simulink library "libMdl_ImuDataCorrector"  (R2019b)
settings: Solver=VariableStepAuto  StartTime=0.0  StopTime=10.0  RelTol=1e-3
undefined symbols (not defined in the file): f_euler_ma_time, imu_lever_arm, sample_time
libraries: libMdl_transformVect x2, libMdl_crossProdMat x2, simulink x1
settings Model: Creator=Hanno  LastModifiedBy=wint_hn

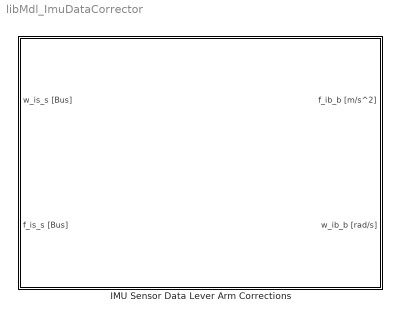
== system libMdl_ImuDataCorrector ==
  IMU Sensor Data Lever Arm Corrections : Subsystem  TreatAsAtomicUnit=on  SystemSampleTime=mv_sample_time  mask(IMU Sensor Data Corrections){mv_lever_arm=imu_lever_arm, mv_mounting_attitude=[1;0;0;0], mv_enable_euler_correction=on, mv_euler_ma_time=f_euler_ma_time, mv_sample_time=sample_time}
      mask prompts: mv_lever_arm "Lever Arm:"; mv_mounting_attitude "Mounting Attitude:"; mv_enable_euler_correction "Enable Euler Correction"; mv_euler_ma_time "Moving Av. Window for Euler Correction:"; mv_sample_time "Sample Time:"
      mask help:
      | Lever Arm: Lever Arm Vector 'leverarm_s_b' in meters describing the mounting position of the sensor with respect to the body frame.
      |
      | Mountin Attitude: Quaternion 'q_s_b' describing the mounting attitude of the sensor with respect to the body frame.
      mask Display:
      | if mv_enable_euler_correction
      |     euler_str = 'on';
      | else
      |     euler_str = 'off';
      | end % if
      | 
      | str1 = sprintf('\\color{black}{\\bfIMU Data Correction}\n\n');
      | str2 = sprintf('Euler Correction: %s\n',euler_str);
      | str3 = sprintf('Euler MA Time: %0.2f\n',mv_euler_ma_time);
      | str4 = sprintf('Sample Time: %0.3f',mv_sample_time);
      | 
      | str = [str1,str2,str3,str4];
      | 
      | text( 0.5,0.5, ...
      |       str, ...
      |       'horizontalAlignment', 'center', ...
      |       'texmode','on' ...
      |     )

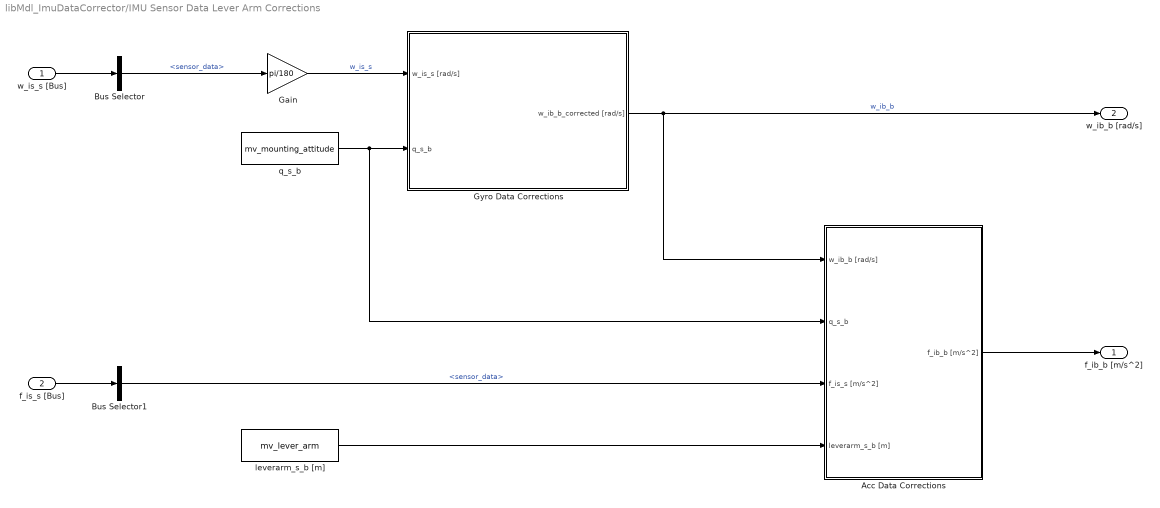
== system libMdl_ImuDataCorrector/IMU Sensor Data Lever Arm Corrections ==
  w_is_s [Bus] : Inport
  f_is_s [Bus] : Inport  Port=2
  Acc Data Corrections : Subsystem
  Bus Selector : BusSelector  OutputSignals=sensor_data
  Bus Selector1 : BusSelector  OutputSignals=sensor_data
  Gain : Gain  Gain=pi/180
      settings: AttributesFormatString=deg2rad
  Gyro Data Corrections : Subsystem
  leverarm_s_b [m] : Constant  Value=mv_lever_arm
  q_s_b : Constant  Value=mv_mounting_attitude
  f_ib_b [m/s^2] : Outport  VectorParamsAs1DForOutWhenUnconnected=off
  w_ib_b [rad/s] : Outport  Port=2  VectorParamsAs1DForOutWhenUnconnected=off
  wires:
  Gyro Data Corrections/1(w_ib_b_corrected [rad/s]) -> w_ib_b [rad/s]/1, Acc Data Corrections/1(w_ib_b [rad/s])  "w_ib_b"
  f_is_s [Bus]/1 -> Bus Selector1/1
  Acc Data Corrections/1(f_ib_b [m/s^2]) -> f_ib_b [m/s^2]/1
  w_is_s [Bus]/1 -> Bus Selector/1
  q_s_b/1 -> Acc Data Corrections/2(q_s_b), Gyro Data Corrections/2(q_s_b)
  leverarm_s_b [m]/1 -> Acc Data Corrections/4(leverarm_s_b [m])
  Bus Selector/1 -> Gain/1  "<sensor_data>"
  Gain/1 -> Gyro Data Corrections/1(w_is_s [rad/s])  "w_is_s"
  Bus Selector1/1 -> Acc Data Corrections/3(f_is_s [m/s^2])  "<sensor_data>"

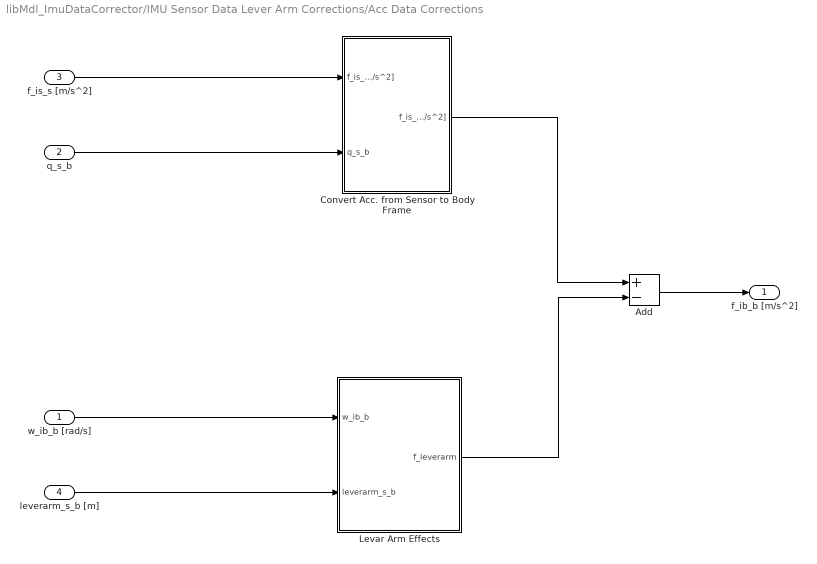
== system libMdl_ImuDataCorrector/IMU Sensor Data Lever Arm Corrections/Acc Data Corrections ==
  w_ib_b [rad/s] : Inport
  q_s_b : Inport  Port=2
  f_is_s [m/s^2] : Inport  Port=3
  leverarm_s_b [m] : Inport  Port=4
  Add : Sum  Inputs=+-
  Convert Acc. from Sensor to Body Frame : Subsystem
  Levar Arm Effects : Subsystem
  f_ib_b [m/s^2] : Outport  VectorParamsAs1DForOutWhenUnconnected=off
  wires:
  Levar Arm Effects/1(f_leverarm) -> Add/2
  f_is_s [m/s^2]/1 -> Convert Acc. from Sensor to Body Frame/1(f_is_s [m/s^2])
  q_s_b/1 -> Convert Acc. from Sensor to Body Frame/2(q_s_b)
  leverarm_s_b [m]/1 -> Levar Arm Effects/2(leverarm_s_b)
  w_ib_b [rad/s]/1 -> Levar Arm Effects/1(w_ib_b)
  Convert Acc. from Sensor to Body Frame/1(f_is_b [m/s^2]) -> Add/1
  Add/1 -> f_ib_b [m/s^2]/1

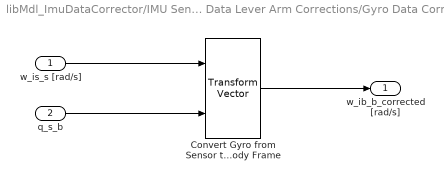
== system libMdl_ImuDataCorrector/IMU Sensor Data Lever Arm Corrections/Gyro Data Corrections ==
  w_is_s [rad/s] : Inport
  q_s_b : Inport  Port=2
  Convert Gyro from Sensor to Body Frame : libMdl_transformVect/Transform Vector  SystemSampleTime=-1  Latency=0  AutoFrameSizeCalculation=off
  w_ib_b_corrected [rad/s] : Outport  VectorParamsAs1DForOutWhenUnconnected=off
  wires:
  Convert Gyro from Sensor to Body Frame/1 -> w_ib_b_corrected [rad/s]/1
  q_s_b/1 -> Convert Gyro from Sensor to Body Frame/2
  w_is_s [rad/s]/1 -> Convert Gyro from Sensor to Body Frame/1

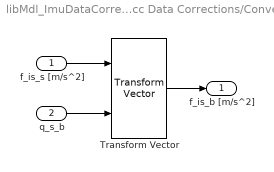
== system libMdl_ImuDataCorrector/IMU Sensor Data Lever Arm Corrections/Acc Data Corrections/Convert Acc. from Sensor to Body Frame ==
  f_is_s [m/s^2] : Inport
  q_s_b : Inport  Port=2
  Transform Vector : libMdl_transformVect/Transform Vector  SystemSampleTime=-1  Latency=0  AutoFrameSizeCalculation=off
  f_is_b [m/s^2] : Outport  VectorParamsAs1DForOutWhenUnconnected=off
  wires:
  f_is_s [m/s^2]/1 -> Transform Vector/1
  q_s_b/1 -> Transform Vector/2
  Transform Vector/1 -> f_is_b [m/s^2]/1

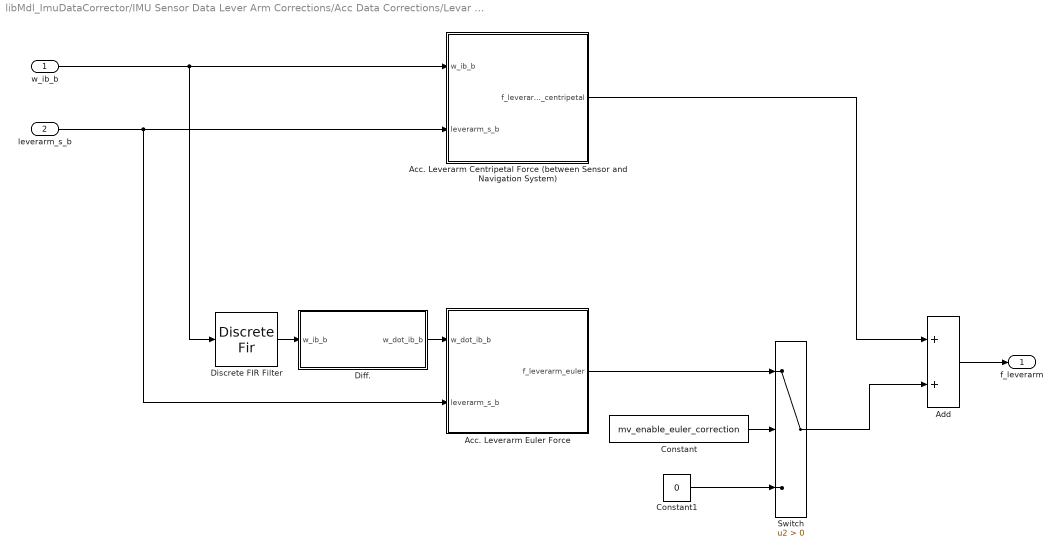
== system libMdl_ImuDataCorrector/IMU Sensor Data Lever Arm Corrections/Acc Data Corrections/Levar Arm Effects ==
  w_ib_b : Inport
  leverarm_s_b : Inport  Port=2
  Acc. Leverarm Centripetal Force (between Sensor and Navigation System) : Subsystem
  Acc. Leverarm Euler Force : Subsystem
  Add : Sum
  Constant : Constant  Value=mv_enable_euler_correction
  Constant1 : Constant  Value=0
  Diff. : Subsystem
  Discrete FIR Filter : DiscreteFir  Coefficients=ones(1,ceil(mv_euler_ma_time/sample_time)) * 1/ceil(mv_euler_ma_time/sample_time)
  Switch : Switch  Criteria=u2 > Threshold
  f_leverarm : Outport  VectorParamsAs1DForOutWhenUnconnected=off
  wires:
  Constant1/1 -> Switch/3
  Acc. Leverarm Euler Force/1(f_leverarm_euler) -> Switch/1
  Constant/1 -> Switch/2
  Switch/1 -> Add/2
  w_ib_b/1 -> Discrete FIR Filter/1, Acc. Leverarm Centripetal Force (between Sensor and Navigation System)/1(w_ib_b)
  Diff./1(w_dot_ib_b) -> Acc. Leverarm Euler Force/1(w_dot_ib_b)
  leverarm_s_b/1 -> Acc. Leverarm Euler Force/2(leverarm_s_b), Acc. Leverarm Centripetal Force (between Sensor and Navigation System)/2(leverarm_s_b)
  Add/1 -> f_leverarm/1
  Acc. Leverarm Centripetal Force (between Sensor and Navigation System)/1(f_leverarm_centripetal) -> Add/1
  Discrete FIR Filter/1 -> Diff./1(w_ib_b)

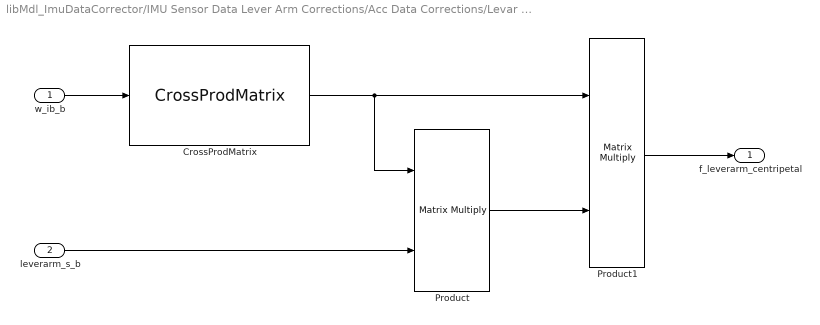
== system libMdl_ImuDataCorrector/IMU Sensor Data Lever Arm Corrections/Acc Data Corrections/Levar Arm Effects/Acc. Leverarm Centripetal Force (between Sensor and Navigation System) ==
  w_ib_b : Inport
  leverarm_s_b : Inport  Port=2
  CrossProdMatrix : libMdl_crossProdMat/CrossProdMatrix  SystemSampleTime=-1  Latency=0  AutoFrameSizeCalculation=off
  Product : Product  Multiplication=Matrix(*)
  Product1 : Product  Multiplication=Matrix(*)
  f_leverarm_centripetal : Outport  VectorParamsAs1DForOutWhenUnconnected=off
  wires:
  CrossProdMatrix/1 -> Product/1, Product1/1
  leverarm_s_b/1 -> Product/2
  Product1/1 -> f_leverarm_centripetal/1
  Product/1 -> Product1/2
  w_ib_b/1 -> CrossProdMatrix/1

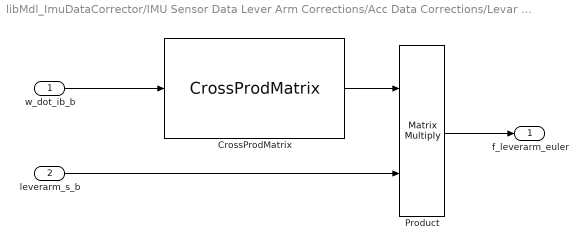
== system libMdl_ImuDataCorrector/IMU Sensor Data Lever Arm Corrections/Acc Data Corrections/Levar Arm Effects/Acc. Leverarm Euler Force ==
  w_dot_ib_b : Inport
  leverarm_s_b : Inport  Port=2
  CrossProdMatrix : libMdl_crossProdMat/CrossProdMatrix  SystemSampleTime=-1  Latency=0  AutoFrameSizeCalculation=off
  Product : Product  Multiplication=Matrix(*)
  f_leverarm_euler : Outport  VectorParamsAs1DForOutWhenUnconnected=off
  wires:
  w_dot_ib_b/1 -> CrossProdMatrix/1
  CrossProdMatrix/1 -> Product/1
  leverarm_s_b/1 -> Product/2
  Product/1 -> f_leverarm_euler/1

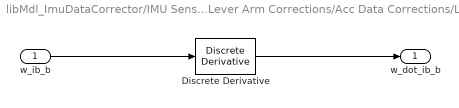
== system libMdl_ImuDataCorrector/IMU Sensor Data Lever Arm Corrections/Acc Data Corrections/Levar Arm Effects/Diff. ==
  w_ib_b : Inport
  Discrete Derivative : simulink/Discrete/Discrete Derivative  gainval=1.0  ICPrevScaledInput=0.0  OutMin=[]  OutMax=[]  OutDataType=fixdt(1, 16)  OutScaling=2^-10  DoSatur=off
  w_dot_ib_b : Outport  VectorParamsAs1DForOutWhenUnconnected=off
  wires:
  Discrete Derivative/1 -> w_dot_ib_b/1
  w_ib_b/1 -> Discrete Derivative/1
